simulink model "testemplanner_cs_old"  (R2020b)
settings: Solver=FixedStepAuto  StartTime=0.0  StopTime=50  FixedStep=1/1000  MaxStep=3  RelTol=1e-3
PreLoadFcn:
  | mbxruntime.callbacks.PreLoadFcn(bdroot);
PostLoadFcn:
  | mbxruntime.callbacks.PostLoadFcn(bdroot);
InitFcn:
  | mbxruntime.callbacks.InitFcn(bdroot);
StartFcn:
  | mbxruntime.callbacks.StartFcn(bdroot);
StopFcn:
  | mbxruntime.callbacks.StopFcn(bdroot);
model workspace (MAT data in the model file):
  mbox_table : object (value not decoded)
  model_closed = 0
  sim_status = 0
values from neighbouring files (symbols this model uses):
  c_factor = 43.75    [emplanner_init.m]
  cf = -175016    [emplanner_init.m]
  cr = -130634    [emplanner_init.m]
  global_path_x = [-8.9703 -7.97092389706 -6.97280725051 -5.97596683104 -4.98040839797 -3.98613358222 -2.99314248891 -2.0014346597 -1.01100942869 -0.0218660539602 0.965996233729 1.95257821297 ... (3001 elements, 3001x1)]    [global_path.mat]
  global_path_y = [9.935 9.935 9.935 9.935 9.935 9.935 9.935 9.935 9.935 9.935 9.935 9.935 ... (3001 elements, 3001x1)]    [global_path.mat]
  KD_PID_distance = 0.0    (= 0)    [emplanner_init.m]
  KD_PID_speed = 0    [emplanner_init.m]
  KI_PID_distance = 0.0    (= 0)    [emplanner_init.m]
  KI_PID_speed = 0    [emplanner_init.m]
  KP_PID_distance = 0.5    [emplanner_init.m]
  KP_PID_speed = 1.8    [emplanner_init.m]
  la = 1.265    [emplanner_init.m]
  lb = 2.947-1.265    (= 1.682)    [emplanner_init.m]
  LQR_K1 = k(:,1)'    [emplanner_init.m]
  LQR_K2 = k(:,2)'    [emplanner_init.m]
  LQR_K3 = k(:,3)'    [emplanner_init.m]
  LQR_K4 = k(:,4)'    [emplanner_init.m]
  m = 2020    [emplanner_init.m]
  rack_displacement = [-39.14 , -37.2 , -35.29 , -33.43 , -31.6 , -29.81 , -28.06 , -26.34 , -24.66 ,      -23.01 , -21.38 , -19.79 , -18.23 , -16.69 , -15.18 , -13.7 , -12.23 , -10.8 , -9.38 , -7.98 ,     -6.61 , -5.25 , -3.91 , -2.59 , -1.29 , 0 , 1.27 , 2.54 , 3.78 , 5.02 , 6.24 , 7.46 , 8.66 ,      9.86 , 11.05 , 12.24 , 13.41 , 14.59 , 15.76 , 16.92 , 18.09 , 19.25 , 20.42 , 21.59 , 22.76 ,      23.93 , 25.11 , 26 ...(+26 chars)    [emplanner_init.m]
  right_wheel_ground = [-70 ,-67.2 , -64.4 , -61.6 , -58.8 , -56 , -53.2 , -50.4 , -47.6 , -44.8 , -42 ,      -39.2 , -36.4 , -33.6 , -30.8 , -28 , -25.2 , -22.4 , -19.6 , -16.8 , -14 , -11.2 , -8.4 , -5.6 ,      -2.8 , 0 , 2.8 , 5.6 , 8.4 , 11.2 , 14 , 16.8 , 19.6 , 22.4 , 25.2 , 28 , 30.8 , 33.6 , 36.4 ,      39.2 , 42 , 44.8 , 47.6 , 50.4 , 53.2 , 56 , 58.8 , 61.6 , 64.4 , 67.2 , 70 ]    [emplanner_init.m]
  vx_break_point = zeros(1,5000)    [emplanner_init.m]
undefined symbols (not defined in the file or in its folder): aubr, DiscIntNeverNeededParam, tablebr, vubr, warningInitialVelocity, x0
libraries: PreScanSimulinkLibrary x33, simulink x19, simulink_extras x10, Solver_SF x1
(part 12 of 12)

== matlab function testemplanner_cs_old/Audi_A8_Sedan_1/decision&planning module/EM planner/MATLAB Function3 ==
  data: dp_speed_s input; dp_speed_t input; qp_speed_s input; qp_speed_t input; obs_s_in_set input; obs_s_out_set input; obs_t_in_set input; obs_t_out_set input
function  fcn(dp_speed_s,dp_speed_t,qp_speed_s,qp_speed_t,obs_s_in_set,obs_s_out_set,obs_t_in_set,obs_t_out_set)
coder.extrinsic("plot");
cla;
n = length(dp_speed_s);
m = length(obs_s_in_set);
s = length(qp_speed_s);
for i = 1:length(dp_speed_s)
    if isnan(dp_speed_s(i))
        n = i -1;
        break;
    end
end
for i = 1:length(qp_speed_s)
    if isnan(qp_speed_s(i))
        s = i -1;
        break;
    end
end

plot(dp_speed_t(1:n),dp_speed_s(1:n),'r')
plot(qp_speed_t(1:s),qp_speed_s(1:s),'b')
hold on
axis([-1 10 -10 50]);
for i = 1:m
    if isnan(obs_s_in_set(i))
        continue;
    end
    point_t = [obs_t_in_set(i),obs_t_out_set(i)];
    point_s = [obs_s_in_set(i),obs_s_out_set(i)];
    plot(point_t,point_s)
end

== matlab function testemplanner_cs_old/Audi_A8_Sedan_1/decision&planning module/referenceline provider/MATLAB Function1 ==
  data: path_x input; path_heading output; path_y input; path_kappa output
function [path_heading,path_kappa] = fcn(path_x,path_y)
%该函数将计算path的切线方向与x轴的夹角和曲率
%输入：path_x,y路径坐标
%输出：path_heading kappa路径的heading和曲率
%原理：heading = actan(dy/dx);
%      kappa = dheading/ds
%      ds = (dx^2 + dy^2)^0.5

dx = diff(path_x);
dy = diff(path_y);
%对dx,dy做中点欧拉法，使用四象限反正切计算角度
dx_pre = [dx(1);dx];
dx_after = [dx;dx(end)];
dx_final = (dx_pre + dx_after) / 2;

dy_pre = [dy(1);dy];
dy_after = [dy;dy(end)];
dy_final = (dy_pre + dy_after) / 2;

ds_final = sqrt(dx_final.^2 + dy_final.^2);
path_heading = atan2(dy_final,dx_final);

dheading = diff(path_heading);
dheading_pre = [dheading(1);dheading];
dheading_after = [dheading;dheading(end)];
dheading_final = (dheading_pre + dheading_after) / 2;
path_kappa = sin(dheading_final) ./ ds_final;
